simulink model "motor_power_model"  (R2026a)
settings: Solver=VariableStepAuto
undefined symbols (not defined in the file): eta_table, rpm_bp, torque_bp
settings Model: Creator=braym  LastModifiedBy=braym

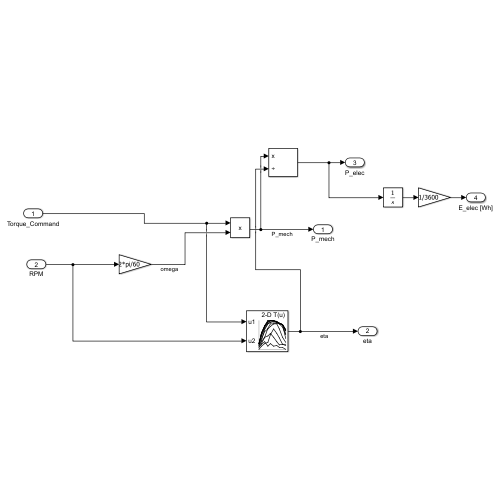
[thumbnail: Simulink's stored preview of the top-level diagram]
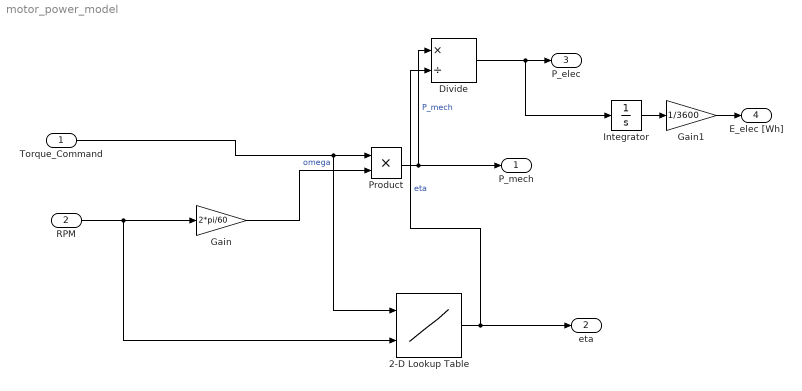
== system motor_power_model ==
  Torque_Command : Inport
  RPM : Inport  Port=2
  2-D Lookup Table : Lookup_n-D  BreakpointsForDimension1=torque_bp  BreakpointsForDimension2=rpm_bp  Table=eta_table  ExtrapMethod=Clip  InternalRulePriority=Speed  RndMeth=Simplest
      settings: InputPortMap=u0,u1
  Divide : Product  Inputs=*/
  Gain : Gain  Gain=2*pi/60
  Gain1 : Gain  Gain=1/3600
  Integrator : Integrator
  Product : Product
  P_mech : Outport
  eta : Outport  Port=2
  P_elec : Outport  Port=3
  E_elec [Wh] : Outport  Port=4
  wires:
  2-D Lookup Table/1 -> Divide/2, eta/1  "eta"
  Gain1/1 -> E_elec [Wh]/1
  RPM/1 -> 2-D Lookup Table/2, Gain/1
  Integrator/1 -> Gain1/1
  Gain/1 -> Product/2  "omega"
  Torque_Command/1 -> 2-D Lookup Table/1, Product/1
  Divide/1 -> Integrator/1, P_elec/1
  Product/1 -> Divide/1, P_mech/1  "P_mech"
